simulink model "exp3"  (R2020b)
settings: Solver=VariableStepAuto  StartTime=0.0  StopTime=10  RelTol=1e-3
libraries: simulink x1
settings Model: Creator=suryanshshukla  LastModifiedBy=suryanshshukla

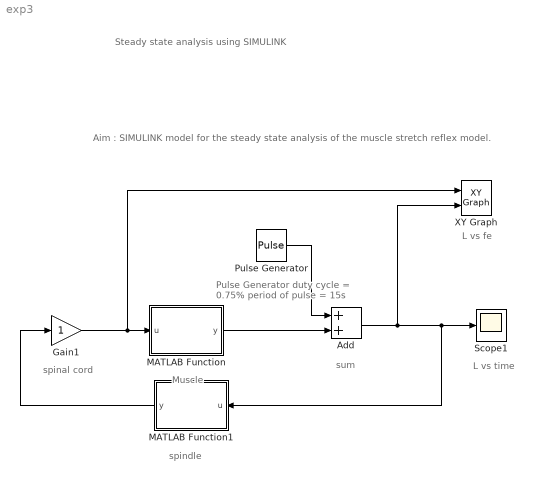
== system exp3 ==
  note: Muscle
  note: spindle
  note: spinal cord
  note: Pulse Generator
      | duty cycle = 0.75%
      | period of pulse = 15s
  note: sum
  note: L vs fe
  note: L vs time
  note: Aim : SIMULINK model for the steady state analysis of the muscle stretch reflex model.
  note: Steady state analysis using SIMULINK
  Add : Sum
  Gain1 : Gain
  MATLAB Function : MATLAB Function  TreatAsAtomicUnit=on
  MATLAB Function1 : MATLAB Function  TreatAsAtomicUnit=on
  Pulse Generator : DiscretePulseGenerator  PulseType=Time based  Period=15  PulseWidth=5
  Scope1 : Scope
  XY Graph : simulink/Sinks/XY Graph  xmin=0.4  xmax=1  ymin=0.4  ymax=1  st=-1
  wires:
  MATLAB Function/1(y) -> Add/2
  Gain1/1 -> XY Graph/1, MATLAB Function/1(u)
  Add/1 -> XY Graph/2, Scope1/1, MATLAB Function1/1(u)
  MATLAB Function1/1(y) -> Gain1/1
  Pulse Generator/1 -> Add/1

== matlab function exp3/MATLAB Function ==
  data: u input; y output
function y = fcn(u)
y= 1 - u^5/(0.5^5 + u^5);

== matlab function exp3/MATLAB Function1 ==
  data: u input; y output
function y = fcn(u)
y= 0.6*u*exp(0.5*u);
